simulink model "embeddedC"  (Simulink 8.5)
settings: Solver=FixedStepDiscrete  StartTime=0.0  StopTime=10.0  FixedStep=1.0  RelTol=1e-3
values from neighbouring files (symbols this model uses):
  cst_param3_system_function = 45    [constants.mat]
  cst_param_system_function = 12    [constants.mat]
settings Model: Creator=arnaud  LastModifiedBy=Teme
settings DataIOCC: SaveFormat=Structure
settings DebuggingCC: SolverPrmCheckMsg=warning  FcnCallInpInsideContextMsg=UseLocalSettings  StrictBusMsg=Warning

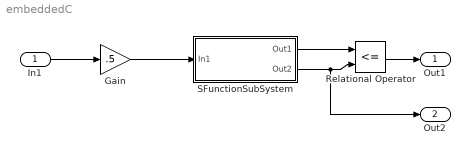
== system embeddedC ==
  In1 : Inport
  Gain : Gain  Gain=.5
  Relational Operator : RelationalOperator  Operator=<=  OutDataTypeStr=boolean
  SFunctionSubSystem : Subsystem  TreatAsAtomicUnit=on
  Out1 : Outport
  Out2 : Outport  Port=2
  wires:
  In1/1 -> Gain/1
  Gain/1 -> SFunctionSubSystem/1(In1)
  SFunctionSubSystem/1(Out1) -> Relational Operator/1
  Relational Operator/1 -> Out1/1
  SFunctionSubSystem/2(Out2) -> Relational Operator/2, Out2/1

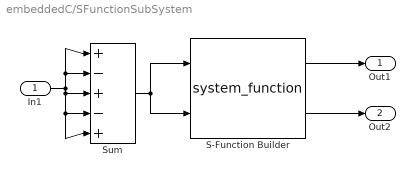
== system embeddedC/SFunctionSubSystem ==
  In1 : Inport
  S-Function Builder : S-Function  InitFcn=try, set_param(gcb,'FunctionName','system_function'), end  FunctionName=system_function  Parameters=cst_param_system_function,boolean(true),cst_param3_system_function  SFunctionModules=system_function_wrapper  WizardData=DataTag0  mask(S-Function Builder){}
      mask help: The S-Function Builder block creates a wrapper C-MEX S-function from your supplied C code with multiple input ports, output ports, and a variable number of scalar, vector, or matrix parameters. The input and output ports can propagate Simulink built-in data types, fixed-point datatypes, complex, frame, 1-D, and 2-D signals. This block also supports discrete and continuous states of type real. You can optionally have the block generate a TLC file to be used with Real-Time Workshop for code generation.
      mask init:
      | val = [[.9  0.75 0.75 1 1 .9 .9 1]',[1 1 0.75 0.75 .9 .9 1 .9]'];try , sys = get_param(gcb,'SfunBuilderFcnName');if isempty(sys), sys = get_param(gcb,'FunctionName'); end,catch, sys = get_param(gcb,'FunctionName'); end
      settings: CopyFcn=set_param(gcbh,'LinkStatus','none')  PreSaveFcn=try, set_param(gcb,'FunctionName','system_function'), end  OpenFcn=sfunctionwizard(gcbh)
      mask Display: plot(val(:,1),val(:,2)),disp(sys), port_label('input',1,'u0'), port_label('input',2,'u1'), port_label('output',1,'y0'), port_label('output',2,'y1')
  Sum : Sum  Inputs=+|-+|-+
  Out1 : Outport
  Out2 : Outport  Port=2
  wires:
  S-Function Builder/1 -> Out1/1
  S-Function Builder/2 -> Out2/1
  Sum/1 -> S-Function Builder/1, S-Function Builder/2
  In1/1 -> Sum/5, Sum/4, Sum/3, Sum/1, Sum/2
